simulink library "vmc"  (R2021b)
settings: Solver=VariableStepAuto  StartTime=0.0  StopTime=10.0  RelTol=1e-3
undefined symbols (not defined in the file): AVMC_ACCDeltaTqGradeGn_X_deg, AVMC_ACCDeltaTqIGain4OVRD_X_kph, AVMC_ACCDeltaTqIGain4OVRD_Y_mps2, AVMC_ACCDeltaTqIGain_X_kph, AVMC_ACCDeltaTqIGain_Y_mps2, AVMC_ACCDeltaTqPGain_X_kph, AVMC_ACCDeltaTqPGain_Y_kph, AVMC_ACCGradeofst_X_G, AVMC_ACCGradeofst_Y_pct, AVMC_ACCLoSpdTqLoLim4JP_X_kph, AVMC_ACCLoSpdTqLoLim4JP_Y_deg, AVMC_ACCLoSpdTqLowerLim_X_kph, AVMC_ACCLoSpdTqLowerLim_Y_deg, AVMC_ACCReqAccelGain_X_mps2, AVMC_ACCReqAccelGain_Y_enum, AVMC_ADSPosGFBDeltaTq_X_kph, AVMC_ADSPosGFBDeltaTq_Y_mps2, AVMC_AggressJerkPCT4AT_X_kph, AVMC_AggressJerkPCT_X_kph, AVMC_AggressLimitPCT4AT_X_kph, AVMC_AggressLimitPCT_X_kph, AVMC_DECGradeofst_X_G, AVMC_DECGradeofst_Y_pct, AVMC_DISCDeltaTqIGain_X_kph, AVMC_DISCDeltaTqIGain_Y_mps2, AVMC_DISCDeltaTqPGain_X_kph, AVMC_DISCDeltaTqPGain_Y_kph, AVMC_EPSForceSelect_X_enum, AVMC_EPSForceSelect_Y_enum, AVMC_EPSForceSelectD21_X_enum, AVMC_EPSForceSelectD21_Y_enum, AVMC_ESCRegenOut_X_kph, AVMC_ESCRegenOut_Y_Deg, AVMC_ESCRegenOutEnSpd_X_Deg, AVMC_EstPitchSlopeTs_X_kph, AVMC_GradeCompFlt_X_kph, AVMC_GyroYBandLo_X_Gps, AVMC_HoldResTq_X_kph, AVMC_ISOAccLimit_X_mps, AVMC_ISODecLimit_X_mps, AVMC_ISOJerk_X_mps, AVMC_LatESCRegenOut_X_kph, AVMC_LatESCRegenOut_Y_Deg, AVMC_LongAccDeadZone_X_kph, AVMC_LongAccFiltTsforP2_X_Gps, AVMC_MCPresBaseTq_X_bar, AVMC_MSAPedalOvrd_X_kph, AVMC_MSASpdBand_X_kph, AVMC_MSATqDownEndTq_X_kph, AVMC_MSATqDownTime_X_kph, AVMC_NegZCHoldTq_X_kph, AVMC_OPDDisSlideRate_X_Deg, AVMC_OVRD2ActSR2FCMCMD_X_mps2, AVMC_PedalTqRWhlRatio_X_Nm, AVMC_PedalTqRWhlRatio_Y_gps, AVMC_PedalTqRWhlSlipGain_X_rat, AVMC_PedalTqRWhlSlipGain_Y_kph, AVMC_PedalTqRWhSTRGGain_X_deg, AVMC_PedalTqRWhSTRGGain_Y_kph, AVMC_PosZCHoldTq_X_kph ... (+593)
libraries: hcu_lib x143, simulink x96, tqr x4, $bdroot x1, simulink_extras x1
(part 5 of 17)

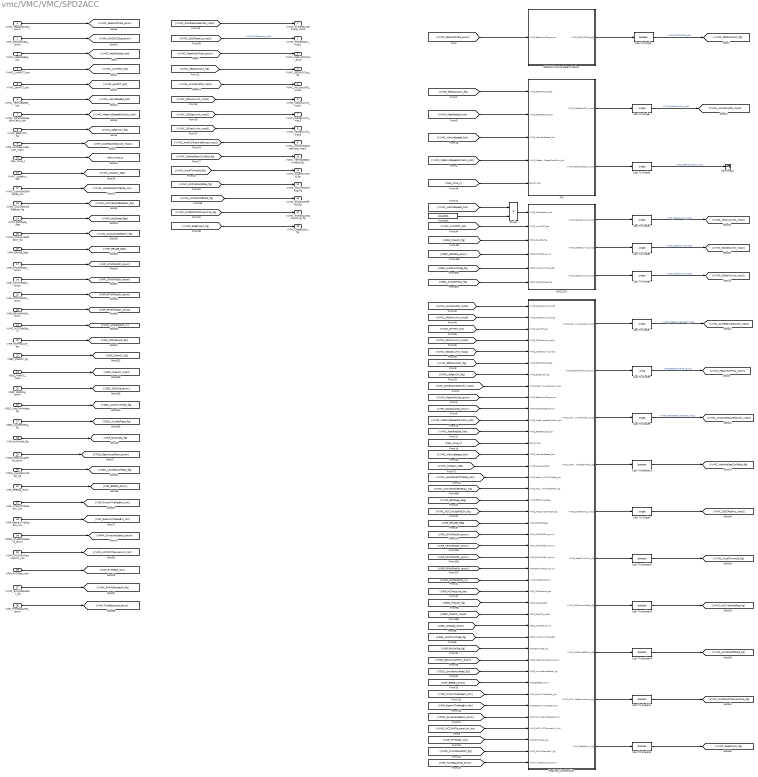
== system vmc/VMC/VMC/SPD2ACC ==
  VVMC_FeatArbitrSta_enum : Inport
  VINP_ADASACCSta_enum : Inport  Port=2
  VVMC_FeatReqSpd_kph : Inport  Port=3
  VVMC_LimitPCT_pct : Inport  Port=4
  VVMC_JerkPCT_pct : Inport  Port=5
  VVMC_VehicleSpeed_kph : Inport  Port=6
  VVMC_MeterIndSpeedForCalcu_kph : Inport  Port=7
  VVMC_SafetyCtrl_flg : Inport  Port=8
  VINP_ACCRequiredAccel_mps2 : Inport  Port=9
  task_time_s : Inport  Port=10
  VVMC_LongAcc_Gps : Inport  Port=11
  VVMC_LastADASWhlTqReq_Nm : Inport  Port=12
  VVMC_ACCVehHoldReqRaw_flg : Inport  Port=13
  VVMC_EstSlope_Deg : Inport  Port=14
  VVMC_ACCLowSpdTqCtrl_flg : Inport  Port=15
  VINP_GRADE_Deg : Inport  Port=16
  VINP_LFWhlRotDir_enum : Inport  Port=17
  VINP_LRWhlRotDir_enum : Inport  Port=18
  VINP_RFWhlRotDir_enum : Inport  Port=19
  VINP_RRWhlRotDir_enum : Inport  Port=20
  VVMC_ACCObjDist_m : Inport  Port=21
  VINP_MCPressure_bar : Inport  Port=22
  VDSC_PreACC_flg : Inport  Port=23
  VDSC_PreACC_mps2 : Inport  Port=24
  VDSC_DISCSta_enum : Inport  Port=25
  VDSC_AutoTurnMode_flg : Inport  Port=26
  VDSC_AccDecResp_flg : Inport  Port=27
  VINP_BrkSwSta_flg : Inport  Port=28
  VTQD_GearActualPosn_enum : Inport  Port=29
  VTQD_LowIdleAccPedal_flg : Inport  Port=30
  VINP_EPBSta_enum : Inport  Port=31
  VINP_FrntAxlTrqReqBrk_Nm : Inport  Port=32
  VINP_RearAxlTrqReqBrk_Nm : Inport  Port=33
  VPMM_DrivetrainSelect_enum : Inport  Port=34
  VVMC_ACCWhlTqLowerLim_Nm : Inport  Port=35
  VINP_RrTMSpd_rpm : Inport  Port=36
  VVMC_RrWhlStandstill_flg : Inport  Port=37
  VINP_TimeGapLevel_enum : Inport  Port=38
  Cast To Boolean{1..4} (4 alike) : DataTypeConversion  OutDataTypeStr=boolean
  Cast To Single : DataTypeConversion  OutDataTypeStr=boolean
  Cast To Single{1..7,9} (8 alike) : DataTypeConversion  OutDataTypeStr=single
  Cast To Single10 : DataTypeConversion  OutDataTypeStr=boolean
  Cast To Single11 : DataTypeConversion  OutDataTypeStr=boolean
  Cast To Single8 : DataTypeConversion  OutDataTypeStr=uint8
  Constant : Constant  Value=KPH2MPS
  Divide : Product  Inputs=**
  ISO22179 : Subsystem
  PID : Subsystem
  Required_Acceleration : Subsystem
  SPD2ACC Active Determination : Subsystem
  Terminator : Terminator
  VVMC_ACCRequiredAccel_mps2 : Outport
  VVMC_DISCReqAcc_mps2 : Outport  Port=2
  VVMC_FeatArbitrFinal_enum : Outport  Port=3
  VVMC_SPD2ACCAct_flg : Outport  Port=4
  VVMC_AccCalcuPID_mps2 : Outport  Port=5
  VVMC_ISOAccLimit_mps2 : Outport  Port=6
  VVMC_ISODecLimit_mps2 : Outport  Port=7
  VVMC_ISOJerkLimit_mps3 : Outport  Port=8
  VVMC_ActACCRequiredAccel_mps2 : Outport  Port=9
  VVMC_VehHoldDecCtrlHEnd_flg : Outport  Port=10
  VVMC_AccelTurnHold_flg : Outport  Port=11
  VVMC_ACCVehHoldReq_flg : Outport  Port=12
  VVMC_ACCShutOffHold_flg : Outport  Port=13
  VVMC_OVRD2ActRampActive_flg : Outport  Port=14
  VVMC_ReqBrkJoin_flg : Outport  Port=15
  wires:
  [VPMM_DrivetrainSelect_enum] -> Required_Acceleration/37(VPMM_DrivetrainSelect_enum)
  VPMM_DrivetrainSelect_enum/1 -> [VPMM_DrivetrainSelect_enum]
  [VINP_FrntAxlTrqReqBrk_Nm] -> Required_Acceleration/35(VINP_FrntAxlTrqReqBrk_Nm)
  [VINP_RearAxlTrqReqBrk_Nm] -> Required_Acceleration/36(VINP_RearAxlTrqReqBrk_Nm)
  VINP_RearAxlTrqReqBrk_Nm/1 -> [VINP_RearAxlTrqReqBrk_Nm]
  VINP_FrntAxlTrqReqBrk_Nm/1 -> [VINP_FrntAxlTrqReqBrk_Nm]
  [task_time_s] -> PID/5(task_time_s)
  [VVMC_OVRD2ActRampActive_flg] -> VVMC_OVRD2ActRampActive_flg/1
  Required_Acceleration/9(VVMC_OVRD2ActRampActive_flg) -> Cast To Single11/1
  Cast To Single11/1 -> [VVMC_OVRD2ActRampActive_flg]
  [VVMC_ACCShutOffHold_flg] -> VVMC_ACCShutOffHold_flg/1
  [VVMC_ACCVehHoldReq_flg] -> VVMC_ACCVehHoldReq_flg/1
  [VVMC_AccelTurnHold_flg] -> VVMC_AccelTurnHold_flg/1
  Cast To Boolean4/1 -> [VVMC_ACCShutOffHold_flg]
  Cast To Boolean3/1 -> [VVMC_ACCVehHoldReq_flg]
  Cast To Boolean2/1 -> [VVMC_AccelTurnHold_flg]
  Required_Acceleration/6(VVMC_AccelTurnHold_flg) -> Cast To Boolean2/1
  Required_Acceleration/7(VVMC_ACCVehHoldReq_flg) -> Cast To Boolean3/1
  Required_Acceleration/8(VVMC_ACCShutOffHold_flg) -> Cast To Boolean4/1
  VTQD_GearActualPosn_enum/1 -> [VTQD_GearActualPosn_enum]
  VINP_EPBSta_enum/1 -> [VINP_EPBSta_enum]
  VINP_BrkSwSta_flg/1 -> [VINP_BrkSwSta_flg]
  VTQD_LowIdleAccPedal_flg/1 -> [VTQD_LowIdleAccPedal_flg]
  [VINP_EPBSta_enum] -> Required_Acceleration/34(VINP_EPBSta_enum)
  [VTQD_LowIdleAccPedal_flg] -> Required_Acceleration/33(VTQD_LowIdleAccPedal_flg)
  [VTQD_GearActualPosn_enum] -> Required_Acceleration/32(VTQD_GearActualPosn_enum)
  [VINP_BrkSwSta_flg] -> Required_Acceleration/31(VINP_BrkSwSta_flg)
  VDSC_PreACC_mps2/1 -> [VDSC_PreACC_mps2]
  VDSC_PreACC_flg/1 -> [VDSC_PreACC_flg]
  VDSC_DISCSta_enum/1 -> [VDSC_DISCSta_enum]
  VDSC_AutoTurnMode_flg/1 -> [VDSC_AutoTurnMode_flg]
  VDSC_AccDecResp_flg/1 -> [VDSC_AccDecResp_flg]
  [VDSC_AutoTurnMode_flg] -> Required_Acceleration/30(VDSC_AutoTurnMode_flg)
  [VDSC_DISCSta_enum] -> Required_Acceleration/29(VDSC_DISCSta_enum)
  [VDSC_PreACC_mps2] -> Required_Acceleration/28(VDSC_PreACC_mps2)
  [VDSC_PreACC_flg] -> Required_Acceleration/27(VDSC_PreACC_flg)
  [VDSC_AccDecResp_flg] -> ISO22179/6(VDSC_AccDecResp_flg)
  [VDSC_AutoTurnMode_flg] -> ISO22179/5(VDSC_AutoTurnMode_flg)
  [VDSC_DISCSta_enum] -> ISO22179/4(VDSC_DISCSta_enum)
  [VDSC_PreACC_flg] -> ISO22179/3(VDSC_PreACC_flg)
  Constant/1 -> Divide/2
  [VVMC_VehicleSpeed_kph] -> Divide/1
  Divide/1 -> ISO22179/1(VVMC_VehSpeed_mps)
  [VVMC_FeatReqSpd_kph] -> PID/2(VVMC_FeatReqSpd_kph)
  Cast To Single3/1 -> [VVMC_DISCReqAcc_mps2]
  Required_Acceleration/5(VVMC_DISCReqAcc_mps2) -> Cast To Single3/1
  [VINP_MCPressure_bar] -> Required_Acceleration/26(VINP_MCPressure_bar)
  VINP_MCPressure_bar/1 -> [VINP_MCPressure_bar]
  [VVMC_ACCObjDist_m] -> Required_Acceleration/25(VVMC_ACCObjDist_m)
  VVMC_ACCObjDist_m/1 -> [VVMC_ACCObjDist_m]
  [VINP_LFWhlRotDir_enum] -> Required_Acceleration/21(VINP_LFWhlRotDir_enum)
  [VINP_LRWhlRotDir_enum] -> Required_Acceleration/22(VINP_LRWhlRotDir_enum)
  [VINP_RFWhlRotDir_enum] -> Required_Acceleration/23(VINP_RFWhlRotDir_enum)
  [VINP_RRWhlRotDir_enum] -> Required_Acceleration/24(VINP_RRWhlRotDir_enum)
  VINP_RRWhlRotDir_enum/1 -> [VINP_RRWhlRotDir_enum]
  VINP_LFWhlRotDir_enum/1 -> [VINP_LFWhlRotDir_enum]
  VINP_RFWhlRotDir_enum/1 -> [VINP_RFWhlRotDir_enum]
  VINP_LRWhlRotDir_enum/1 -> [VINP_LRWhlRotDir_enum]
  [VINP_GRADE_Deg] -> Required_Acceleration/20(VINP_GRADE_Deg)
  VINP_GRADE_Deg/1 -> [VINP_GRADE_Deg]
  [VVMC_ACCLowSpdTqCtrl_flg] -> Required_Acceleration/19(VVMC_ACCLowSpdTqCtrl_flg)
  VVMC_ACCLowSpdTqCtrl_flg/1 -> [VVMC_ACCLowSpdTqCtrl_flg]
  [VVMC_VehHoldDecCtrlHEnd_flg] -> VVMC_VehHoldDecCtrlHEnd_flg/1
  Cast To Boolean1/1 -> [VVMC_VehHoldDecCtrlHEnd_flg]
  Required_Acceleration/4(VVMC_VehHoldDecCtrlHEnd_flg) -> Cast To Boolean1/1
  [VVMC_EstSlope_Deg] -> Required_Acceleration/18(VVMC_EstSlope_Deg)
  VVMC_EstSlope_Deg/1 -> [VVMC_EstSlope_Deg]
  [VVMC_ACCVehHoldReqRaw_flg] -> Required_Acceleration/17(VVMC_ACCVehHoldReqRaw_flg)
  VVMC_ACCVehHoldReqRaw_flg/1 -> [VVMC_ACCVehHoldReqRaw_flg]
  [VVMC_ActACCRequiredAccel_mps2] -> VVMC_ActACCRequiredAccel_mps2/1
  VVMC_LastADASWhlTqReq_Nm/1 -> [VVMC_LastADASWhlTqReq_Nm]
  Required_Acceleration/3(VVMC_ActACCRequiredAccel_mps2) -> Cast To Single9/1
  Cast To Single9/1 -> [VVMC_ActACCRequiredAccel_mps2]  "VVMC_ActACCRequiredAccel_mps2"
  [VVMC_LastADASWhlTqReq_Nm] -> Required_Acceleration/16(VVMC_LastADASWhlTqReq_Nm)
  VVMC_LongAcc_Gps/1 -> [VVMC_LongAcc_Gps]
  [VVMC_LongAcc_Gps] -> Required_Acceleration/15(VVMC_LongAcc_Gps)
  [VVMC_VehicleSpeed_kph] -> Required_Acceleration/14(VVMC_VehicleSpeed_kph)
  [VVMC_ISODecLimit_mps2] -> Required_Acceleration/5(VVMC_ISODecLimit_mps2)
  [VVMC_ISOAccLimit_mps2] -> Required_Acceleration/4(VVMC_ISOAccLimit_mps2)
  [VVMC_AccCalcuPID_mps2] -> Required_Acceleration/1(VVMC_AccCalcuPID_mps2)
  [VVMC_ISOJerkLimit_mps3] -> Required_Acceleration/2(VVMC_ISOJerkLimit_mps3)
  [VVMC_JerkPCT_pct] -> Required_Acceleration/3(VVMC_JerkPCT_pct)
  VVMC_FeatReqSpd_kph/1 -> [VVMC_FeatReqSpd_kph]
  VVMC_JerkPCT_pct/1 -> [VVMC_JerkPCT_pct]
  VVMC_LimitPCT_pct/1 -> [VVMC_LimitPCT_pct]
  VVMC_MeterIndSpeedForCalcu_kph/1 -> [VVMC_MeterIndSpeedForCalcu_kph]
  VVMC_FeatArbitrSta_enum/1 -> [VVMC_FeatArbitrSta_enum]
  [VVMC_FeatArbitrSta_enum] -> SPD2ACC Active Determination/1(VVMC_FeatArbitrSta_enum)
  SPD2ACC Active Determination/1(VVMC_SPD2ACCAct_flg) -> Cast To Single/1
  [VVMC_LimitPCT_pct] -> ISO22179/2(VVMC_LimitPCT_pct)
  ISO22179/1(VVMC_ISOAccLimit_mps2) -> Cast To Single4/1
  ISO22179/2(VVMC_ISODecLimit_mps2) -> Cast To Single5/1
  ISO22179/3(VVMC_ISOJerkLimit_mps3) -> Cast To Single6/1
  [VVMC_SPD2ACCAct_flg] -> PID/1(VVMC_SPD2ACCAct_flg)
  [VVMC_MeterIndSpeedForCalcu_kph] -> PID/4(VVMC_MeterIndSpeedForCalcu_kph)
  PID/1(VVMC_AccCalcuPID_mps2) -> Cast To Single1/1
  PID/2(VVMC_MeterSpdCalcu_mps) -> Cast To Single2/1
  [VVMC_SPD2ACCAct_flg] -> Required_Acceleration/6(VVMC_SPD2ACCAct_flg)
  Required_Acceleration/1("VVMC_ACCRequiredAccel_mps2 ") -> Cast To Single7/1
  [VVMC_ACCRequiredAccel_mps2] -> VVMC_ACCRequiredAccel_mps2/1
  Cast To Single/1 -> [VVMC_SPD2ACCAct_flg]  "VVMC_SPD2ACCAct_flg"
  Cast To Single1/1 -> [VVMC_AccCalcuPID_mps2]  "VVMC_AccCalcuPID_mps2"
  Cast To Single2/1 -> Terminator/1  "VVMC_MeterSpdCalcu_mps"
  Cast To Single4/1 -> [VVMC_ISOAccLimit_mps2]  "VVMC_ISOAccLimit_mps2"
  Cast To Single5/1 -> [VVMC_ISODecLimit_mps2]  "VVMC_ISODecLimit_mps2"
  Cast To Single6/1 -> [VVMC_ISOJerkLimit_mps3]  "VVMC_ISOJerkLimit_mps3"
  Cast To Single7/1 -> [VVMC_ACCRequiredAccel_mps2]  "VVMC_ACCRequiredAccel_mps2"
  [VVMC_SafetyCtrl_flg] -> Required_Acceleration/7(VVMC_SafetyCtrl_flg)
  VVMC_SafetyCtrl_flg/1 -> [VVMC_SafetyCtrl_flg]
  VINP_ACCRequiredAccel_mps2/1 -> [VINP_ACCRequiredAccel_mps2]
  [VINP_ACCRequiredAccel_mps2] -> Required_Acceleration/8(VINP_ACCRequiredAccel_mps2)
  [VVMC_FeatArbitrSta_enum] -> Required_Acceleration/9(VVMC_FeatArbitrSta_enum)
  Required_Acceleration/2(VVMC_FeatArbitrFinal_enum) -> Cast To Single8/1
  Cast To Single8/1 -> [VVMC_FeatArbitrFinal_enum]  "VVMC_FeatArbitrFinal_enum"
  [VVMC_FeatArbitrFinal_enum] -> VVMC_FeatArbitrFinal_enum/1
  [VVMC_DISCReqAcc_mps2] -> VVMC_DISCReqAcc_mps2/1  "VVMC_DISCReqAcc_mps2"
  VINP_ADASACCSta_enum/1 -> [VINP_ADASACCSta_enum]
  [VINP_ADASACCSta_enum] -> Required_Acceleration/10(VINP_ADASACCSta_enum)
  [VVMC_MeterIndSpeedForCalcu_kph] -> Required_Acceleration/11(VVMC_MeterIndSpeedForCalcu_kph)
  [VVMC_FeatReqSpd_kph] -> Required_Acceleration/12(VVMC_FeatReqSpd_kph)
  [VVMC_SPD2ACCAct_flg] -> VVMC_SPD2ACCAct_flg/1
  [VVMC_AccCalcuPID_mps2] -> VVMC_AccCalcuPID_mps2/1
  [VVMC_ISOAccLimit_mps2] -> VVMC_ISOAccLimit_mps2/1
  [VVMC_ISODecLimit_mps2] -> VVMC_ISODecLimit_mps2/1
  [VVMC_ISOJerkLimit_mps3] -> VVMC_ISOJerkLimit_mps3/1
  VVMC_VehicleSpeed_kph/1 -> [VVMC_VehicleSpeed_kph]
  [VVMC_VehicleSpeed_kph] -> PID/3(VVMC_VehicleSpeed_kph)
  task_time_s/1 -> [task_time_s]
  [task_time_s] -> Required_Acceleration/13(task_time_s)
  Required_Acceleration/10(VVMC_ReqBrkJoin_flg) -> Cast To Single10/1
  Cast To Single10/1 -> [VVMC_ReqBrkJoin_flg]
  [VVMC_ReqBrkJoin_flg] -> VVMC_ReqBrkJoin_flg/1
  VVMC_ACCWhlTqLowerLim_Nm/1 -> [VVMC_ACCWhlTqLowerLim_Nm]
  [VVMC_ACCWhlTqLowerLim_Nm] -> Required_Acceleration/38(VVMC_ACCWhlTqLowerLim_Nm)
  [VINP_RrTMSpd_rpm] -> Required_Acceleration/39(VINP_RrTMSpd_rpm)
  VINP_RrTMSpd_rpm/1 -> [VINP_RrTMSpd_rpm]
  VVMC_RrWhlStandstill_flg/1 -> [VVMC_RrWhlStandstill_flg]
  [VVMC_RrWhlStandstill_flg] -> Required_Acceleration/40(VVMC_RrWhlStandstill_flg)
  VINP_TimeGapLevel_enum/1 -> [VINP_TimeGapLevel_enum]
  [VINP_TimeGapLevel_enum] -> Required_Acceleration/41(VINP_TimeGapLevel_enum)

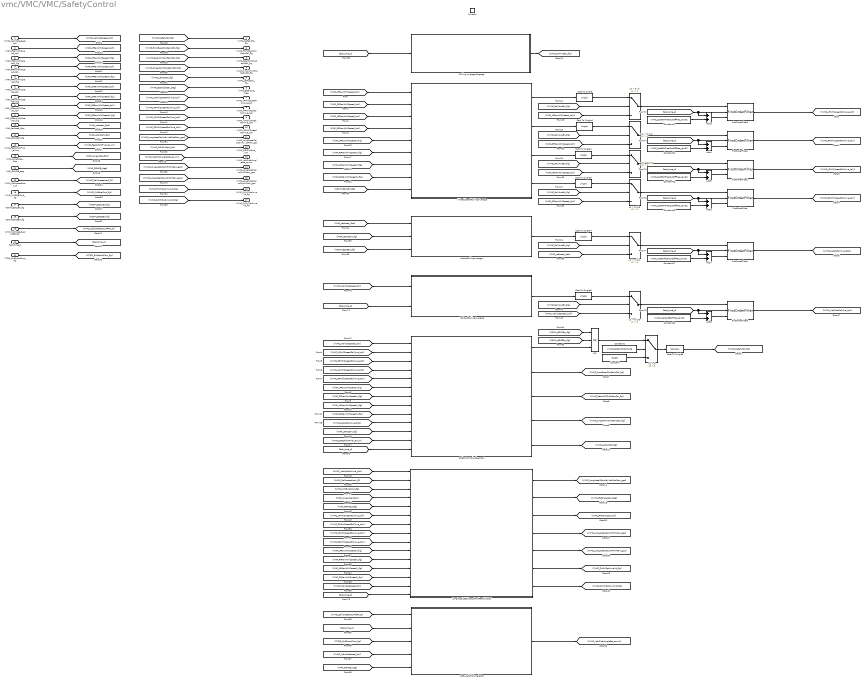
== system vmc/VMC/VMC/SafetyControl ==
  VVMC_VehicleSpeed_kph : Inport
  VINP_LFRawWhlSpeed_kph : Inport  Port=2
  VINP_LFRawWhlSpeedV_flg : Inport  Port=3
  VINP_RFRawWhlSpeed_kph : Inport  Port=4
  VINP_RFRawWhlSpeedV_flg : Inport  Port=5
  VINP_LRRawWhlSpeed_kph : Inport  Port=6
  VINP_LRRawWhlSpeedV_flg : Inport  Port=7
  VINP_RRRawWhlSpeed_kph : Inport  Port=8
  VINP_RRRawWhlSpeedV_flg : Inport  Port=9
  VINP_LatAccel_Gps : Inport  Port=10
  VINP_LatAccelV_flg : Inport  Port=11
  VVMC_FeatArbitrFinal_enum : Inport  Port=12
  VINP_LongAccel_Gps : Inport  Port=13
  VINP_GRADE_deg : Inport  Port=14
  VVMC_CalibratedAccX_G : Inport  Port=15
  VVMC_IMUEnaCmd_flg : Inport  Port=16
  VDDM_ESC1Err_flg : Inport  Port=17
  VDDM_ESC5Err_flg : Inport  Port=18
  VVMC_CalibratedAccXAftRA_G : Inport  Port=19
  task_time_s : Inport  Port=20
  VTQD_ExtDoorAllow_flg : Inport  Port=21
  function : TriggerPort  TriggerType=function-call  VariantControl=(inherit)
  ADB_VehPitchAngleSta : Subsystem
  Add{3..8} (6 alike) : Sum
  Cast To Single{,1..4,8} (6 alike) : DataTypeConversion  OutDataTypeStr=single
  Cast To Single5 : DataTypeConversion  OutDataTypeStr=boolean
  Constant : Constant  Value=FALSE
  Constant1 : Constant  Value=KVMC_SafetyCtrlSWC_flg
  Constant{11..13,15} (4 alike) : Constant  Value=KVMC_SpdBWFilterCutOffFreq_raw32
  Constant17 : Constant  Value=KVMC_AccBWFilterCutOffFreq_raw32
  Constant23 : Constant  Value=KVMC_VehSpdBWFilter_raw32
  FirstOrderFilter{,1..4,6} (6 alike) : hcu_lib/Basic_Blocks/FirstOrderFilter
  LatAccRollingAverage : Subsystem
  LongAccel_EstSlope_FrontRearSlipSpd : Subsystem
  OR : Logic  Operator=OR  Inputs=3  AllPortsSameDT=off  OutDataTypeStr=boolean
  Rolling Average Engage : Subsystem
  SafetyControlJudgement : Subsystem
  VehSpdRollingAverage : Subsystem
  WheelSpeedRollingAverage : Subsystem
  u2 > 0 : Switch  Criteria=u2 > Threshold
  u2 > 0 (1){,1..4,6} (6 alike) : Switch  Criteria=u2 > Threshold
  VVMC_SafetyCtrl_flg : Outport
  VVMC_FrontRearSlipRatioCtrl_flg : Outport  Port=2
  VVMC_RearWhlSlipRatioCtrl_flg : Outport  Port=3
  VVMC_SingleWhlSlipRatioCtrl_flg : Outport  Port=4
  VVMC_LatAccCtrl_flg : Outport  Port=5
  VVMC_EstSlope_Deg : Outport  Port=6
  VVMC_LFWhlSpeedRollAve_kph : Outport  Port=7
  VVMC_RFWhlSpeedRollAve_kph : Outport  Port=8
  VVMC_LRWhlSpeedRollAve_kph : Outport  Port=9
  VVMC_RRWhlSpeedRollAve_kph : Outport  Port=10
  VVMC_LongAccelCalcuByVehSpdRaw_gps : Outport  Port=11
  VVMC_FrRrSlipSpd_kph : Outport  Port=12
  VVMC_VehPitchAngleSta_enum : Outport  Port=13
  VVMC_LongAccelCalcuFrWhlRaw_gps : Outport  Port=14
  VVMC_LongAccelCalcuRrWhlRaw_gps : Outport  Port=15
  VVMC_FrWhlSpdInvalid_flg : Outport  Port=16
  VVMC_RrWhlSpdInvalid_flg : Outport  Port=17
  wires:
  [VVMC_VehPitchAngleSta_enum] -> VVMC_VehPitchAngleSta_enum/1
  VTQD_ExtDoorAllow_flg/1 -> [VTQD_ExtDoorAllow_flg]
  task_time_s/1 -> [task_time_s]
  VVMC_CalibratedAccXAftRA_G/1 -> [VVMC_CalibratedAccXAftRA_G]
  OR/1 -> u2 > 0/1
  [VDDM_ESC1Err_flg] -> OR/1
  [VDDM_ESC5Err_flg] -> OR/2
  [VDDM_ESC5Err_flg] -> LatAccRollingAverage/3(VDDM_ESC5Err_flg)
  [VDDM_ESC1Err_flg] -> WheelSpeedRollingAverage/9(VDDM_ESC1Err_flg)
  VDDM_ESC5Err_flg/1 -> [VDDM_ESC5Err_flg]
  VDDM_ESC1Err_flg/1 -> [VDDM_ESC1Err_flg]
  [VINP_LatAccelV_flg] -> LatAccRollingAverage/2(VINP_LatAccelV_flg)
  [VINP_RRRawWhlSpeedV_flg] -> WheelSpeedRollingAverage/8(VINP_RRRawWhlSpeedV_flg)
  [VINP_LRRawWhlSpeedV_flg] -> WheelSpeedRollingAverage/7(VINP_LRRawWhlSpeedV_flg)
  [VINP_RFRawWhlSpeedV_flg] -> WheelSpeedRollingAverage/6(VINP_RFRawWhlSpeedV_flg)
  [VINP_LFRawWhlSpeedV_flg] -> WheelSpeedRollingAverage/5(VINP_LFRawWhlSpeedV_flg)
  VVMC_IMUEnaCmd_flg/1 -> [VVMC_IMUEnaCmd_flg]
  VVMC_CalibratedAccX_G/1 -> [VVMC_CalibratedAccX_G]
  [VVMC_FrRrSlipSpd_kph] -> VVMC_FrRrSlipSpd_kph/1
  [VVMC_LongAccelCalcuByVehSpdRaw_gps] -> VVMC_LongAccelCalcuByVehSpdRaw_gps/1  "VVMC_LongAccelCalcuByVehSpd_gps"
  VehSpdRollingAverage/1(VVMC_VehSpdRollAveRaw_kph) -> Cast To Single8/1
  FirstOrderFilter6/1 -> [VVMC_VehSpdRollAve_kph]  "VVMC_VehSpdRollAve_kph"
  [VVMC_RollAveEn_flg] -> u2 > 0 (1)6/2
  [VVMC_VehicleSpeed_kph] -> u2 > 0 (1)6/3
  u2 > 0 (1)6/1 -> FirstOrderFilter6/1
  Cast To Single8/1 -> u2 > 0 (1)6/1
  [task_time_s] -> FirstOrderFilter6/2, Add8/1
  Constant23/1 -> Add8/2
  Add8/1 -> FirstOrderFilter6/3
  [VVMC_VehicleSpeed_kph] -> VehSpdRollingAverage/1(VVMC_VehicleSpeed_kph)
  [VVMC_LFWhlSpeedRollAve_kph] -> VVMC_LFWhlSpeedRollAve_kph/1  "VVMC_LFWhlSpeedRollAve_kph"
  [VVMC_RFWhlSpeedRollAve_kph] -> VVMC_RFWhlSpeedRollAve_kph/1  "VVMC_RFWhlSpeedRollAve_kph"
  [VVMC_LRWhlSpeedRollAve_kph] -> VVMC_LRWhlSpeedRollAve_kph/1  "VVMC_LRWhlSpeedRollAve_kph"
  [VVMC_RRWhlSpeedRollAve_kph] -> VVMC_RRWhlSpeedRollAve_kph/1  "VVMC_RRWhlSpeedRollAve_kph"
  [VVMC_EstSlopeCal_Deg] -> VVMC_EstSlope_Deg/1
  VINP_GRADE_deg/1 -> [VINP_GRADE_deg]
  VINP_LongAccel_Gps/1 -> [VINP_LongAccel_Gps]
  u2 > 0 (1)4/1 -> FirstOrderFilter4/1
  [task_time_s] -> Add7/1, FirstOrderFilter4/2
  Constant17/1 -> Add7/2
  Add7/1 -> FirstOrderFilter4/3
  [VINP_LatAccel_Gps] -> u2 > 0 (1)4/3
  Cast To Single4/1 -> u2 > 0 (1)4/1
  [VVMC_RollAveEn_flg] -> u2 > 0 (1)4/2
  Add6/1 -> FirstOrderFilter/3
  Constant15/1 -> Add6/2
  Add5/1 -> FirstOrderFilter1/3
  Constant13/1 -> Add5/2
  Add4/1 -> FirstOrderFilter2/3
  Constant12/1 -> Add4/2
  Constant11/1 -> Add3/2
  Add3/1 -> FirstOrderFilter3/3
  [task_time_s] -> Add6/1, FirstOrderFilter/2
  [task_time_s] -> FirstOrderFilter1/2, Add5/1
  [task_time_s] -> Add4/1, FirstOrderFilter2/2
  [task_time_s] -> FirstOrderFilter3/2, Add3/1
  [VVMC_RollAveEn_flg] -> u2 > 0 (1)2/2
  Cast To Single3/1 -> u2 > 0 (1)3/1
  u2 > 0 (1)3/1 -> FirstOrderFilter/1
  Cast To Single1/1 -> u2 > 0 (1)1/1
  Cast To Single2/1 -> u2 > 0 (1)2/1
  [VVMC_RollAveEn_flg] -> u2 > 0 (1)1/2
  u2 > 0 (1)1/1 -> FirstOrderFilter2/1
  [VINP_RRRawWhlSpeed_kph] -> u2 > 0 (1)3/3
  Cast To Single/1 -> u2 > 0 (1)/1
  [VINP_LFRawWhlSpeed_kph] -> u2 > 0 (1)/3
  [VVMC_RollAveEn_flg] -> u2 > 0 (1)/2
  [VVMC_RollAveEn_flg] -> u2 > 0 (1)3/2
  [VINP_LRRawWhlSpeed_kph] -> u2 > 0 (1)2/3
  [VINP_RFRawWhlSpeed_kph] -> u2 > 0 (1)1/3
  u2 > 0 (1)/1 -> FirstOrderFilter3/1
  u2 > 0 (1)2/1 -> FirstOrderFilter1/1
  VINP_RFRawWhlSpeedV_flg/1 -> [VINP_RFRawWhlSpeedV_flg]
  Constant/1 -> u2 > 0/3
  FirstOrderFilter1/1 -> [VVMC_LRWhlSpeedRollAve_kph]  "VVMC_LRWhlSpeedRollAve_kph"
  [VVMC_RFWhlSpeedRollAve_kph] -> SafetyControlJudgement/3(VVMC_RFWhlSpeedRollAve_kph)
  VINP_RFRawWhlSpeed_kph/1 -> [VINP_RFRawWhlSpeed_kph]
  Cast To Single5/1 -> [VVMC_SafetyCtrl_flg]  "VVMC_SafetyCtrl_flg"
  [VVMC_FrontRearSlipRatioCtrl_flg] -> VVMC_FrontRearSlipRatioCtrl_flg/1
  [VVMC_LFWhlSpeedRollAve_kph] -> SafetyControlJudgement/2(VVMC_LFWhlSpeedRollAve_kph)
  FirstOrderFilter2/1 -> [VVMC_RFWhlSpeedRollAve_kph]  "VVMC_RFWhlSpeedRollAve_kph"
  [VVMC_SafetyCtrl_flg] -> VVMC_SafetyCtrl_flg/1
  VVMC_VehicleSpeed_kph/1 -> [VVMC_VehicleSpeed_kph]
  VINP_LRRawWhlSpeedV_flg/1 -> [VINP_LRRawWhlSpeedV_flg]
  [VVMC_VehicleSpeed_kph] -> SafetyControlJudgement/1(VVMC_VehicleSpeed_kph)
  VVMC_FeatArbitrFinal_enum/1 -> [VVMC_FeatArbitrFinal_enum]
  [VINP_LRRawWhlSpeedV_flg] -> SafetyControlJudgement/8(VINP_LRRawWhlSpeedV_flg)
  [VINP_RRRawWhlSpeedV_flg] -> SafetyControlJudgement/9(VINP_RRRawWhlSpeedV_flg)
  SafetyControlJudgement/1(VVMC_SafetyCtrl_flg) -> OR/3
  [VVMC_FeatArbitrFinal_enum] -> SafetyControlJudgement/12(VVMC_FeatArbitrFinal_enum)
  VINP_LFRawWhlSpeedV_flg/1 -> [VINP_LFRawWhlSpeedV_flg]
  [VINP_LFRawWhlSpeed_kph] -> WheelSpeedRollingAverage/1(VINP_LFRawWhlSpeed_kph)
  VINP_LatAccelV_flg/1 -> [VINP_LatAccelV_flg]
  SafetyControlJudgement/3(VVMC_RearWhlSlipRatioCtrl_flg) -> [VVMC_RearWhlSlipRatioCtrl_flg]
  WheelSpeedRollingAverage/3(VVMC_LRWhlSpeedRollAveRaw_kph) -> Cast To Single2/1
  [VVMC_RRWhlSpeedRollAve_kph] -> SafetyControlJudgement/5(VVMC_RRWhlSpeedRollAve_kph)
  [VINP_RRRawWhlSpeed_kph] -> WheelSpeedRollingAverage/4(VINP_RRRawWhlSpeed_kph)
  [VVMC_LRWhlSpeedRollAve_kph] -> SafetyControlJudgement/4(VVMC_LRWhlSpeedRollAve_kph)
  VINP_RRRawWhlSpeedV_flg/1 -> [VINP_RRRawWhlSpeedV_flg]
  [VVMC_RearWhlSlipRatioCtrl_flg] -> VVMC_RearWhlSlipRatioCtrl_flg/1
  u2 > 0/1 -> Cast To Single5/1
  FirstOrderFilter4/1 -> [VVMC_LatAccRollAve_Gps]  "VVMC_LatAccRollAve_Gps"
  VINP_LRRawWhlSpeed_kph/1 -> [VINP_LRRawWhlSpeed_kph]
  Constant1/1 -> u2 > 0/2
  [VINP_RFRawWhlSpeedV_flg] -> SafetyControlJudgement/7(VINP_RFRawWhlSpeedV_flg)
  [VVMC_LatAccCtrl_flg] -> VVMC_LatAccCtrl_flg/1
  SafetyControlJudgement/4(VVMC_SingleWhlSlipRatioCtrl_flg) -> [VVMC_SingleWhlSlipRatioCtrl_flg]
  WheelSpeedRollingAverage/1(VVMC_LFWhlSpeedRollAveRaw_kph) -> Cast To Single/1
  VINP_LatAccel_Gps/1 -> [VINP_LatAccel_Gps]
  LatAccRollingAverage/1(VVMC_LatAccRollAveRaw_Gps) -> Cast To Single4/1
  [VINP_LatAccel_Gps] -> LatAccRollingAverage/1(VINP_LatAccel_Gps)
  VINP_RRRawWhlSpeed_kph/1 -> [VINP_RRRawWhlSpeed_kph]
  [VINP_LFRawWhlSpeedV_flg] -> SafetyControlJudgement/6(VINP_LFRawWhlSpeedV_flg)
  [VINP_LatAccelV_flg] -> SafetyControlJudgement/11(VINP_LatAccelV_flg)
  FirstOrderFilter3/1 -> [VVMC_LFWhlSpeedRollAve_kph]  "VVMC_LFWhlSpeedRollAve_kph"
  WheelSpeedRollingAverage/2(VVMC_RFWhlSpeedRollAveRaw_kph) -> Cast To Single1/1
  [VINP_RFRawWhlSpeed_kph] -> WheelSpeedRollingAverage/2(VINP_RFRawWhlSpeed_kph)
  SafetyControlJudgement/5(VVMC_LatAccCtrl_flg) -> [VVMC_LatAccCtrl_flg]
  SafetyControlJudgement/2(VVMC_FrontRearSlipRatioCtrl_flg) -> [VVMC_FrontRearSlipRatioCtrl_flg]
  VINP_LFRawWhlSpeed_kph/1 -> [VINP_LFRawWhlSpeed_kph]
  [VVMC_SingleWhlSlipRatioCtrl_flg] -> VVMC_SingleWhlSlipRatioCtrl_flg/1
  [VVMC_LatAccRollAve_Gps] -> SafetyControlJudgement/10(VVMC_LatAccRollAve_Gps)
  FirstOrderFilter/1 -> [VVMC_RRWhlSpeedRollAve_kph]  "VVMC_RRWhlSpeedRollAve_kph"
  [VINP_LRRawWhlSpeed_kph] -> WheelSpeedRollingAverage/3(VINP_LRRawWhlSpeed_kph)
  WheelSpeedRollingAverage/4(VVMC_RRWhlSpeedRollAveRaw_kph) -> Cast To Single3/1
  Rolling Average Engage/1(VVMC_RollAveEn_flg) -> [VVMC_RollAveEn_flg]
  [VVMC_VehSpdRollAve_kph] -> LongAccel_EstSlope_FrontRearSlipSpd/1(VVMC_VehSpdRollAve_kph)
  [VVMC_CalibratedAccX_G] -> LongAccel_EstSlope_FrontRearSlipSpd/2(VVMC_CalibratedAccX_G)
  [VVMC_IMUEnaCmd_flg] -> LongAccel_EstSlope_FrontRearSlipSpd/3(VVMC_IMUEnaCmd_flg)
  [VINP_LongAccel_Gps] -> LongAccel_EstSlope_FrontRearSlipSpd/4(VINP_LongAccel_Gps)
  [VINP_GRADE_deg] -> LongAccel_EstSlope_FrontRearSlipSpd/5(VINP_GRADE_deg)
  [VVMC_LFWhlSpeedRollAve_kph] -> LongAccel_EstSlope_FrontRearSlipSpd/6(VVMC_LFWhlSpeedRollAve_kph)
  [VVMC_RFWhlSpeedRollAve_kph] -> LongAccel_EstSlope_FrontRearSlipSpd/7(VVMC_RFWhlSpeedRollAve_kph)
  [VVMC_LRWhlSpeedRollAve_kph] -> LongAccel_EstSlope_FrontRearSlipSpd/8(VVMC_LRWhlSpeedRollAve_kph)
  [VVMC_RRWhlSpeedRollAve_kph] -> LongAccel_EstSlope_FrontRearSlipSpd/9(VVMC_RRWhlSpeedRollAve_kph)
  [VINP_LFRawWhlSpeedV_flg] -> LongAccel_EstSlope_FrontRearSlipSpd/10(VINP_LFRawWhlSpeedV_flg)
  [VINP_RFRawWhlSpeedV_flg] -> LongAccel_EstSlope_FrontRearSlipSpd/11(VINP_RFRawWhlSpeedV_flg)
  [VINP_LRRawWhlSpeedV_flg] -> LongAccel_EstSlope_FrontRearSlipSpd/12(VINP_LRRawWhlSpeedV_flg)
  [VINP_RRRawWhlSpeedV_flg] -> LongAccel_EstSlope_FrontRearSlipSpd/13(VINP_RRRawWhlSpeedV_flg)
  LongAccel_EstSlope_FrontRearSlipSpd/1(VVMC_LongAccelCalcuByVehSpdRaw_gps) -> [VVMC_LongAccelCalcuByVehSpdRaw_gps]
  LongAccel_EstSlope_FrontRearSlipSpd/2(VVMC_EstSlopeCal_Deg) -> [VVMC_EstSlopeCal_Deg]
  LongAccel_EstSlope_FrontRearSlipSpd/3(VVMC_FrRrSlipSpd_kph) -> [VVMC_FrRrSlipSpd_kph]
  ADB_VehPitchAngleSta/1(VVMC_VehPitchAngleSta_enum) -> [VVMC_VehPitchAngleSta_enum]
  [VVMC_CalibratedAccXAftRA_G] -> ADB_VehPitchAngleSta/1(VVMC_CalibratedAccXAftRA_G)
  [task_time_s] -> ADB_VehPitchAngleSta/2(task_time_s)
  [VTQD_ExtDoorAllow_flg] -> ADB_VehPitchAngleSta/3(VTQD_ExtDoorAllow_flg)
  [VVMC_VehicleSpeed_kph] -> ADB_VehPitchAngleSta/4(VVMC_VehicleSpeed_kph)
  [VINP_GRADE_deg] -> ADB_VehPitchAngleSta/5(VINP_GRADE_deg)
  [VVMC_VehicleSpeed_kph] -> LongAccel_EstSlope_FrontRearSlipSpd/14(VVMC_VehicleSpeed_kph)
  [task_time_s] -> VehSpdRollingAverage/2(task_time_s)
  [task_time_s] -> LongAccel_EstSlope_FrontRearSlipSpd/15(task_time_s)
  [task_time_s] -> Rolling Average Engage/1(task_time_s)
  [task_time_s] -> SafetyControlJudgement/13(task_time_s)
  [VVMC_LongAccelCalcuRrWhlRaw_gps] -> VVMC_LongAccelCalcuRrWhlRaw_gps/1
  [VVMC_LongAccelCalcuFrWhlRaw_gps] -> VVMC_LongAccelCalcuFrWhlRaw_gps/1
  LongAccel_EstSlope_FrontRearSlipSpd/4(VVMC_LongAccelCalcuFrWhlRaw_gps) -> [VVMC_LongAccelCalcuFrWhlRaw_gps]
  LongAccel_EstSlope_FrontRearSlipSpd/5(VVMC_LongAccelCalcuRrWhlRaw_gps) -> [VVMC_LongAccelCalcuRrWhlRaw_gps]
  LongAccel_EstSlope_FrontRearSlipSpd/6(VVMC_FrWhlSpdInvalid_flg) -> [VVMC_FrWhlSpdInvalid_flg]
  LongAccel_EstSlope_FrontRearSlipSpd/7(VVMC_RrWhlSpdInvalid_flg) -> [VVMC_RrWhlSpdInvalid_flg]
  [VVMC_FrWhlSpdInvalid_flg] -> VVMC_FrWhlSpdInvalid_flg/1
  [VVMC_RrWhlSpdInvalid_flg] -> VVMC_RrWhlSpdInvalid_flg/1

== system vmc/VMC/VMC/Slide Rate  Calculation ==
  VINP_LFRawWhlSpeed_kph : Inport
  VINP_RFRawWhlSpeed_kph : Inport  Port=2
  VINP_LRRawWhlSpeed_kph : Inport  Port=3
  VINP_RRRawWhlSpeed_kph : Inport  Port=4
  VVMC_VehicleSpeed_kph : Inport  Port=5
  VINP_BrkPedalPos_pct : Inport  Port=6
  VINP_BrkSwSta_flg : Inport  Port=7
  VINP_LongAccel_Gps : Inport  Port=8
  VVMC_LongAcc_Gps : Inport  Port=9
  task_time_s : Inport  Port=10
  VTQD_AfterAvailableTqDemFr_Nm : Inport  Port=11
  VTQD_AfterAvailableTqDemRr_Nm : Inport  Port=12
  VTQD_EquivAccPedalSWSta_flg : Inport  Port=13
  VTQD_GearActualPosn_enum : Inport  Port=14
  VTQD_RegenMode_enum : Inport  Port=15
  VTQD_VehActSpd_kph : Inport  Port=16
  VVMC_EstSlope_Deg : Inport  Port=17
  4Wheel Calculation : Subsystem
  Alternative Wheel Slide Calculation : Subsystem
  Coordination : Subsystem
  Partial Wheel Calculation : Subsystem
  VVMC_RawWhlSpdSlideRate_pct : Outport
  VVMC_LFWhlSpdSlideRate_pct : Outport  Port=2
  VVMC_RFWhlSpdSlideRate_pct : Outport  Port=3
  VVMC_LRWhlSpdSlideRate_pct : Outport  Port=4
  VVMC_RRWhlSpdSlideRate_pct : Outport  Port=5
  VVMC_LF4WhlSpdSlideRate_pct : Outport  Port=6
  VVMC_RF4WhlSpdSlideRate_pct : Outport  Port=7
  VVMC_LR4WhlSpdSlideRate_pct : Outport  Port=8
  VVMC_RR4WhlSpdSlideRate_pct : Outport  Port=9
  VVMC_PredictVehSpd_kph : Outport  Port=10
  VVMC_4WhlSpdSlideRate_pct : Outport  Port=11
  VVMC_ActMaxSlideRate_pct : Outport  Port=12
  VVMC_ActLFSlideRate_pct : Outport  Port=13
  VVMC_ActRFSlideRate_pct : Outport  Port=14
  VVMC_ActLRSlideRate_pct : Outport  Port=15
  VVMC_ActRRSlideRate_pct : Outport  Port=16
  VVMC_AltLWhlSlideRate_pct : Outport  Port=17
  VVMC_AltRWhlSlideRate_pct : Outport  Port=18
  VVMC_AltWhlSlideRate_pct : Outport  Port=19
  wires:
  [VVMC_EstSlope_Deg] -> Coordination/23(VVMC_EstSlope_Deg)
  [VTQD_VehActSpd_kph] -> Coordination/21(VTQD_VehActSpd_kph)
  [VTQD_RegenMode_enum] -> Coordination/22(VTQD_RegenMode_enum)
  VTQD_VehActSpd_kph/1 -> [VTQD_VehActSpd_kph]
  VTQD_RegenMode_enum/1 -> [VTQD_RegenMode_enum]
  VVMC_EstSlope_Deg/1 -> [VVMC_EstSlope_Deg]
  [VINP_LongAccel_Gps] -> 4Wheel Calculation/11(VINP_LongAccel_Gps)
  VINP_LongAccel_Gps/1 -> [VINP_LongAccel_Gps]
  VTQD_GearActualPosn_enum/1 -> [VTQD_GearActualPosn_enum]
  [VTQD_GearActualPosn_enum] -> 4Wheel Calculation/10(VTQD_GearActualPosn_enum)
  [VVMC_RF4WhlSpdSlideRate_pct] -> Coordination/15(VVMC_RF4WhlSpdSlideRate_pct)
  Coordination/2(VVMC_ActLFSlideRate_pct) -> [VVMC_ActLFSlideRate_pct]
  Coordination/5(VVMC_ActRRSlideRate_pct) -> [VVMC_ActRRSlideRate_pct]
  Coordination/1(VVMC_ActMaxSlideRate_pct) -> [VVMC_ActMaxSlideRate_pct]
  [VINP_BrkPedalPos_pct] -> Coordination/3(VINP_BrkPedalPos_pct)
  [VVMC_RRWhlSpdSlideRate_pct] -> Coordination/12(VVMC_RRWhlSpdSlideRate_pct)
  [VVMC_LRWhlSpdSlideRate_pct] -> Coordination/11(VVMC_LRWhlSpdSlideRate_pct)
  [VINP_BrkSwSta_flg] -> Coordination/7(VINP_BrkSwSta_flg)
  [VVMC_PredictVehSpd_kph] -> Coordination/4(VVMC_PredictVehSpd_kph)
  Coordination/4(VVMC_ActLRSlideRate_pct) -> [VVMC_ActLRSlideRate_pct]
  [VTQD_AfterAvailableTqDemRr_Nm] -> Coordination/19(VTQD_AfterAvailableTqDemRr_Nm)
  [VVMC_RawWhlSpdSlideRate_pct] -> Coordination/8(VVMC_RawWhlSpdSlideRate_pct)
  Coordination/3(VVMC_ActRFSlideRate_pct) -> [VVMC_ActRFSlideRate_pct]
  [VVMC_VehicleSpeed_kph] -> Coordination/5(VVMC_VehicleSpeed_kph)
  [VVMC_4WhlSpdSlideRate_pct] -> Coordination/13(VVMC_4WhlSpdSlideRate_pct)
  [VVMC_AllWhlSkid_flg] -> Coordination/18(VVMC_AllWhlSkid_flg)
  [VTQD_EquivAccPedalSWSta_flg] -> Coordination/2(VTQD_EquivAccPedalSWSta_flg)
  [VVMC_RFWhlSpdSlideRate_pct] -> Coordination/10(VVMC_RFWhlSpdSlideRate_pct)
  [VVMC_AltWhlSlideRate_pct] -> Coordination/20(VVMC_AltWhlSlideRate_pct)
  [VTQD_AfterAvailableTqDemFr_Nm] -> Coordination/1(VTQD_AfterAvailableTqDemFr_Nm)
  [VVMC_LFWhlSpdSlideRate_pct] -> Coordination/9(VVMC_LFWhlSpdSlideRate_pct)
  [task_time_s] -> Coordination/6(task_time_s)
  [VVMC_LR4WhlSpdSlideRate_pct] -> Coordination/16(VVMC_LR4WhlSpdSlideRate_pct)
  [VVMC_RR4WhlSpdSlideRate_pct] -> Coordination/17(VVMC_RR4WhlSpdSlideRate_pct)
  [VVMC_LF4WhlSpdSlideRate_pct] -> Coordination/14(VVMC_LF4WhlSpdSlideRate_pct)
  4Wheel Calculation/6(VVMC_4WhlSpdSlideRate_pct) -> [VVMC_4WhlSpdSlideRate_pct]
  4Wheel Calculation/2(VVMC_RF4WhlSpdSlideRate_pct) -> [VVMC_RF4WhlSpdSlideRate_pct]
  [VINP_RFRawWhlSpeed_kph] -> 4Wheel Calculation/2(VINP_RFRawWhlSpeed_kph)
  [VINP_LFRawWhlSpeed_kph] -> 4Wheel Calculation/1(VINP_LFRawWhlSpeed_kph)
  [VINP_RRRawWhlSpeed_kph] -> 4Wheel Calculation/4(VINP_RRRawWhlSpeed_kph)
  [VINP_LRRawWhlSpeed_kph] -> 4Wheel Calculation/3(VINP_LRRawWhlSpeed_kph)
  4Wheel Calculation/5(VVMC_PredictVehSpd_kph) -> [VVMC_PredictVehSpd_kph]
  [VVMC_VehicleSpeed_kph] -> 4Wheel Calculation/7(VVMC_VehicleSpeed_kph)
  [VTQD_AfterAvailableTqDemFr_Nm] -> 4Wheel Calculation/8(VTQD_AfterAvailableTqDemFr_Nm)
  [VTQD_AfterAvailableTqDemRr_Nm] -> 4Wheel Calculation/9(VTQD_AfterAvailableTqDemRr_Nm)
  4Wheel Calculation/4(VVMC_RR4WhlSpdSlideRate_pct) -> [VVMC_RR4WhlSpdSlideRate_pct]
  [VVMC_LongAcc_Gps] -> 4Wheel Calculation/5(VVMC_LongAcc_Gps)
  4Wheel Calculation/7(VVMC_AllWhlSkid_flg) -> [VVMC_AllWhlSkid_flg]
  4Wheel Calculation/1(VVMC_LF4WhlSpdSlideRate_pct) -> [VVMC_LF4WhlSpdSlideRate_pct]
  [task_time_s] -> 4Wheel Calculation/6(task_time_s)
  4Wheel Calculation/3(VVMC_LR4WhlSpdSlideRate_pct) -> [VVMC_LR4WhlSpdSlideRate_pct]
  Partial Wheel Calculation/4(VVMC_LRWhlSpdSlideRate_pct) -> [VVMC_LRWhlSpdSlideRate_pct]
  [VTQD_AfterAvailableTqDemRr_Nm] -> Partial Wheel Calculation/6(VTQD_AfterAvailableTqDemRr_Nm)
  [VINP_RRRawWhlSpeed_kph] -> Partial Wheel Calculation/4(VINP_RRRawWhlSpeed_kph)
  [VINP_LFRawWhlSpeed_kph] -> Partial Wheel Calculation/1(VINP_LFRawWhlSpeed_kph)
  [VTQD_AfterAvailableTqDemFr_Nm] -> Partial Wheel Calculation/5(VTQD_AfterAvailableTqDemFr_Nm)
  [VINP_LRRawWhlSpeed_kph] -> Partial Wheel Calculation/3(VINP_LRRawWhlSpeed_kph)
  [VINP_RFRawWhlSpeed_kph] -> Partial Wheel Calculation/2(VINP_RFRawWhlSpeed_kph)
  Partial Wheel Calculation/1(VVMC_RawWhlSpdSlideRate_pct) -> [VVMC_RawWhlSpdSlideRate_pct]
  Partial Wheel Calculation/3(VVMC_RFWhlSpdSlideRate_pct) -> [VVMC_RFWhlSpdSlideRate_pct]
  Partial Wheel Calculation/5(VVMC_RRWhlSpdSlideRate_pct) -> [VVMC_RRWhlSpdSlideRate_pct]
  Partial Wheel Calculation/2(VVMC_LFWhlSpdSlideRate_pct) -> [VVMC_LFWhlSpdSlideRate_pct]
  [VVMC_AltWhlSlideRate_pct] -> VVMC_AltWhlSlideRate_pct/1
  [VVMC_AltRWhlSlideRate_pct] -> VVMC_AltRWhlSlideRate_pct/1
  [VVMC_AltLWhlSlideRate_pct] -> VVMC_AltLWhlSlideRate_pct/1
  Alternative Wheel Slide Calculation/3(VVMC_AltWhlSlideRate_pct) -> [VVMC_AltWhlSlideRate_pct]
  Alternative Wheel Slide Calculation/2(VVMC_AltRWhlSlideRate_pct) -> [VVMC_AltRWhlSlideRate_pct]
  Alternative Wheel Slide Calculation/1(VVMC_AltLWhlSlideRate_pct) -> [VVMC_AltLWhlSlideRate_pct]
  [VINP_RRRawWhlSpeed_kph] -> Alternative Wheel Slide Calculation/4(VINP_RRRawWhlSpeed_kph)
  [VINP_LRRawWhlSpeed_kph] -> Alternative Wheel Slide Calculation/3(VINP_LRRawWhlSpeed_kph)
  [VINP_RFRawWhlSpeed_kph] -> Alternative Wheel Slide Calculation/2(VINP_RFRawWhlSpeed_kph)
  [VINP_LFRawWhlSpeed_kph] -> Alternative Wheel Slide Calculation/1(VINP_LFRawWhlSpeed_kph)
  VTQD_AfterAvailableTqDemRr_Nm/1 -> [VTQD_AfterAvailableTqDemRr_Nm]
  VVMC_LongAcc_Gps/1 -> [VVMC_LongAcc_Gps]
  [VVMC_4WhlSpdSlideRate_pct] -> VVMC_4WhlSpdSlideRate_pct/1
  [VVMC_ActLFSlideRate_pct] -> VVMC_ActLFSlideRate_pct/1
  [VVMC_LRWhlSpdSlideRate_pct] -> VVMC_LRWhlSpdSlideRate_pct/1
  VINP_LFRawWhlSpeed_kph/1 -> [VINP_LFRawWhlSpeed_kph]
  [VVMC_RawWhlSpdSlideRate_pct] -> VVMC_RawWhlSpdSlideRate_pct/1
  [VVMC_LF4WhlSpdSlideRate_pct] -> VVMC_LF4WhlSpdSlideRate_pct/1
  VINP_LRRawWhlSpeed_kph/1 -> [VINP_LRRawWhlSpeed_kph]
  [VVMC_PredictVehSpd_kph] -> VVMC_PredictVehSpd_kph/1
  [VVMC_ActLRSlideRate_pct] -> VVMC_ActLRSlideRate_pct/1
  VVMC_VehicleSpeed_kph/1 -> [VVMC_VehicleSpeed_kph]
  VINP_RFRawWhlSpeed_kph/1 -> [VINP_RFRawWhlSpeed_kph]
  [VVMC_RR4WhlSpdSlideRate_pct] -> VVMC_RR4WhlSpdSlideRate_pct/1
  [VVMC_ActRFSlideRate_pct] -> VVMC_ActRFSlideRate_pct/1
  [VVMC_LR4WhlSpdSlideRate_pct] -> VVMC_LR4WhlSpdSlideRate_pct/1
  [VVMC_RFWhlSpdSlideRate_pct] -> VVMC_RFWhlSpdSlideRate_pct/1
  [VVMC_ActMaxSlideRate_pct] -> VVMC_ActMaxSlideRate_pct/1
  VINP_RRRawWhlSpeed_kph/1 -> [VINP_RRRawWhlSpeed_kph]
  task_time_s/1 -> [task_time_s]
  [VVMC_RRWhlSpdSlideRate_pct] -> VVMC_RRWhlSpdSlideRate_pct/1
  VINP_BrkPedalPos_pct/1 -> [VINP_BrkPedalPos_pct]
  [VVMC_LFWhlSpdSlideRate_pct] -> VVMC_LFWhlSpdSlideRate_pct/1
  VTQD_EquivAccPedalSWSta_flg/1 -> [VTQD_EquivAccPedalSWSta_flg]
  [VVMC_ActRRSlideRate_pct] -> VVMC_ActRRSlideRate_pct/1
  [VVMC_RF4WhlSpdSlideRate_pct] -> VVMC_RF4WhlSpdSlideRate_pct/1
  VTQD_AfterAvailableTqDemFr_Nm/1 -> [VTQD_AfterAvailableTqDemFr_Nm]
  VINP_BrkSwSta_flg/1 -> [VINP_BrkSwSta_flg]

== system vmc/VMC/VMC/SpeedArbitration ==
  VVMC_VMCCCCtrlAvail_flg : Inport
  VVMC_VMCMSACtrlAvail_flg : Inport  Port=2
  VVMC_VMCACCCtrlAvail_flg : Inport  Port=3
  VVMC_VMCAEBCtrlAvail_flg : Inport  Port=4
  VINP_ADASAEBReq_enum : Inport  Port=5
  VINP_ADASAEBSta_enum : Inport  Port=6
  VDSC_DISCSta_enum : Inport  Port=7
  VINP_ADASACCSta_enum : Inport  Port=8
  VVMC_CCCtrlSta_enum : Inport  Port=9
  VVMC_MSACtrlSta_enum : Inport  Port=10
  VDSC_DISCTargetSpd_kph : Inport  Port=11
  VVMC_FeatSetSpdForCalcu_kph : Inport  Port=12
  VDSC_DISCTurn_flg : Inport  Port=13
  VVMC_MeterIndSpeedForCalcu_kph : Inport  Port=14
  VVMC_VehicleSpeed_kph : Inport  Port=15
  VDSC_AccDecResp_flg : Inport  Port=16
  VDSC_AutoTurnMode_flg : Inport  Port=17
  VVMC_AntiSpdLimSpdEn_flg : Inport  Port=18
  VVMC_AntiLimitSpd_kph : Inport  Port=19
  VDSC_PreACC_flg : Inport  Port=20
  AND : Logic  AllPortsSameDT=off  OutDataTypeStr=boolean
  AND1 : Logic  AllPortsSameDT=off  OutDataTypeStr=boolean
  Cast To Single : DataTypeConversion  OutDataTypeStr=uint8
  Cast To Single1 : DataTypeConversion  OutDataTypeStr=uint8
  Cast To Single2 : DataTypeConversion  OutDataTypeStr=single
  Cast To Single3 : DataTypeConversion  OutDataTypeStr=single
  Cast To Single4 : DataTypeConversion  OutDataTypeStr=single
  Constant : Constant  Value=KVMC_ExternalCtrlSW_flg
  Constant1 : Constant  Value=KVMC_ExternalCtrlSW_flg
  Constant11 : Constant  Value=KVMC_DISCDecCtrlTest_flg
  Constant12 : Constant  Value=ENUM_DISCSTA_ACTIVE
  Constant13 : Constant  Value=HUNDRED
  Constant14 : Constant  Value=KVMC_DISCDecCtrlTest_flg
  Constant15 : Constant  Value=ENUM_DISCSTA_ACTIVE
  Constant16 : Constant  Value=HUNDRED
  Constant2 : Constant  Value=KVMC_ExternalCtrlSW_flg
  Constant3 : Constant  Value=KVMC_ExternalCtrlSta_enum
  Constant4 : Constant  Value=KVMC_ExternalSpeedTarget_kph
  Constant5 : Constant  Value=KVMC_ExternalCtrlAGSV_flg
  Constant6 : Constant  Value=KVMC_AutoTurnJerkHiGain_pct
  Constant7 : Constant  Value=KVMC_AutoTurnLimitHiGain_pct
  Constant8 : Constant  Value=ENUM_FEATSTACFM_MSA
  Constant9 : Constant  Value=ENUM_FEATSTACFM_MSA
  Divide : Product  Inputs=**
  Divide1 : Product  Inputs=**
  Feature Arbitration : Subsystem
  Feature Status Confirm : Subsystem
  OR : Logic  Operator=OR  Inputs=3  AllPortsSameDT=off  OutDataTypeStr=boolean
  OR1 : Logic  Operator=OR  Inputs=3  AllPortsSameDT=off  OutDataTypeStr=boolean
  Relational Operator : RelationalOperator  Operator===  OutDataTypeStr=boolean  RndMeth=Simplest
  Relational Operator1 : RelationalOperator  Operator===  OutDataTypeStr=boolean  RndMeth=Simplest
  Response Gain : Subsystem
  Round : Rounding  Operator=round
  Switch{,1..9} (10 alike) : Switch  Criteria=u2 > Threshold
  VVMC_FeatArbitrSta_enum : Outport
  VVMC_FeatReqSpd_kph : Outport  Port=2
  VVMC_JerkPCT_pct : Outport  Port=3
  VVMC_LimitPCT_pct : Outport  Port=4
  wires:
  [VDSC_PreACC_flg] -> Feature Arbitration/4(VDSC_PreACC_flg)
  [VDSC_PreACC_flg] -> Feature Status Confirm/11(VDSC_PreACC_flg)
  Switch8/1 -> [VVMC_JerkPCT_pct]  "VVMC_JerkPCT_pct"
  AND/1 -> Switch8/2
  OR/1 -> AND/1
  [VDSC_AutoTurnMode_flg] -> OR/3
  Constant11/1 -> AND/2
  Constant12/1 -> Relational Operator/2
  [VDSC_PreACC_flg] -> OR/1
  Constant13/1 -> Switch8/1
  Relational Operator/1 -> OR/2
  [VDSC_DISCSta_enum] -> Relational Operator/1
  Switch9/1 -> [VVMC_LimitPCT_pct]  "VVMC_LimitPCT_pct"
  Constant14/1 -> AND1/2
  Constant16/1 -> Switch9/1
  [VDSC_AutoTurnMode_flg] -> OR1/3
  [VDSC_DISCSta_enum] -> Relational Operator1/1
  Constant15/1 -> Relational Operator1/2
  OR1/1 -> AND1/1
  [VDSC_PreACC_flg] -> OR1/1
  Relational Operator1/1 -> OR1/2
  AND1/1 -> Switch9/2
  VDSC_PreACC_flg/1 -> [VDSC_PreACC_flg]
  VVMC_AntiLimitSpd_kph/1 -> [VVMC_AntiLimitSpd_kph]
  [VDSC_DISCTargetSpd_kph] -> Response Gain/7(VDSC_DISCTargetSpd_kph)
  [VVMC_AntiLimitSpd_kph] -> Switch7/1
  Cast To Single2/1 -> Switch7/3
  [VVMC_AntiSpdLimSpdEn_flg] -> Switch7/2
  Cast To Single1/1 -> Switch6/3
  [VVMC_AntiSpdLimSpdEn_flg] -> Switch6/2
  Constant9/1 -> Switch6/1
  Constant8/1 -> Switch5/1
  Cast To Single/1 -> Switch5/3
  [VVMC_AntiSpdLimSpdEn_flg] -> Switch5/2
  VVMC_AntiSpdLimSpdEn_flg/1 -> [VVMC_AntiSpdLimSpdEn_flg]
  [VDSC_AutoTurnMode_flg] -> Response Gain/6(VDSC_AutoTurnMode_flg)
  VDSC_AutoTurnMode_flg/1 -> [VDSC_AutoTurnMode_flg]
  [VDSC_AccDecResp_flg] -> Switch4/2
  Cast To Single4/1 -> Switch4/3, Divide1/2
  Constant7/1 -> Divide1/1
  Divide1/1 -> Switch4/1
  Divide/1 -> Switch3/1
  Constant6/1 -> Divide/1
  Cast To Single3/1 -> Divide/2, Switch3/3
  [VDSC_AccDecResp_flg] -> Switch3/2
  VDSC_AccDecResp_flg/1 -> [VDSC_AccDecResp_flg]
  [VDSC_DISCTurn_flg] -> Switch2/3
  Constant/1 -> Switch/2
  Constant4/1 -> Switch1/1
  Constant2/1 -> Switch2/2
  Constant3/1 -> Switch/1
  [VDSC_DISCTargetSpd_kph] -> Switch1/3
  Constant5/1 -> Switch2/1
  Constant1/1 -> Switch1/2
  [VDSC_DISCSta_enum] -> Switch/3
  Switch1/1 -> Feature Arbitration/2(VDSC_DISCTargetSpd_kph)
  VINP_ADASAEBSta_enum/1 -> [VINP_ADASAEBSta_enum]
  VDSC_DISCSta_enum/1 -> [VDSC_DISCSta_enum]
  VINP_ADASACCSta_enum/1 -> [VINP_ADASACCSta_enum]
  VVMC_CCCtrlSta_enum/1 -> [VVMC_CCCtrlSta_enum]
  VVMC_MSACtrlSta_enum/1 -> [VVMC_MSACtrlSta_enum]
  VDSC_DISCTargetSpd_kph/1 -> [VDSC_DISCTargetSpd_kph]
  VVMC_FeatSetSpdForCalcu_kph/1 -> [VVMC_FeatSetSpdForCalcu_kph]
  VDSC_DISCTurn_flg/1 -> [VDSC_DISCTurn_flg]
  [VINP_ADASAEBSta_enum] -> Feature Status Confirm/5(VINP_ADASAEBSta_enum)
  Switch/1 -> Feature Status Confirm/6(VDSC_DISCSta_enum)
  [VINP_ADASACCSta_enum] -> Feature Status Confirm/7(VINP_ADASACCSta_enum)
  [VVMC_CCCtrlSta_enum] -> Feature Status Confirm/8(VVMC_CCCtrlSta_enum)
  [VVMC_MSACtrlSta_enum] -> Feature Status Confirm/9(VVMC_MSACtrlSta_enum)
  Feature Status Confirm/1(VVMC_FeatStaConfirm_enum) -> Cast To Single/1
  [VVMC_FeatStaConfirm_enum] -> Feature Arbitration/1(VVMC_FeatStaConfirm_enum)
  [VVMC_FeatSetSpdForCalcu_kph] -> Feature Arbitration/3(VVMC_FeatSetSpdForCalcu_kph)
  Feature Arbitration/1(VVMC_FeatArbitrSta_enum) -> Cast To Single1/1
  Feature Arbitration/2(VVMC_FeatReqSpd_kph) -> Round/1
  [VVMC_FeatArbitrSta_enum] -> VVMC_FeatArbitrSta_enum/1
  [VVMC_FeatReqSpd_kph] -> VVMC_FeatReqSpd_kph/1
  Switch2/1 -> Response Gain/1(VDSC_DISCTurn_flg)
  [VVMC_FeatArbitrSta_enum] -> Response Gain/2(VVMC_FeatArbitrSta_enum)
  Response Gain/2(VVMC_LimitPCT_pct) -> Cast To Single4/1
  Response Gain/1(VVMC_JerkPCT_pct) -> Cast To Single3/1
  [VVMC_LimitPCT_pct] -> VVMC_LimitPCT_pct/1
  [VVMC_JerkPCT_pct] -> VVMC_JerkPCT_pct/1
  Switch5/1 -> [VVMC_FeatStaConfirm_enum]  "VVMC_FeatStaConfirm_enum"
  Switch6/1 -> [VVMC_FeatArbitrSta_enum]  "VVMC_FeatArbitrSta_enum"
  Switch7/1 -> [VVMC_FeatReqSpd_kph]  "VVMC_FeatReqSpd_kph"
  Switch3/1 -> Switch8/3
  Switch4/1 -> Switch9/3
  VVMC_VMCACCCtrlAvail_flg/1 -> [VVMC_VMCACCCtrlAvail_flg]
  VVMC_VMCAEBCtrlAvail_flg/1 -> [VVMC_VMCAEBCtrlAvail_flg]
  [VVMC_VMCACCCtrlAvail_flg] -> Feature Status Confirm/4(VVMC_VMCACCCtrlAvail_flg)
  [VVMC_VMCAEBCtrlAvail_flg] -> Feature Status Confirm/3(VVMC_VMCAEBCtrlAvail_flg)
  VVMC_VMCMSACtrlAvail_flg/1 -> [VVMC_VMCMSACtrlAvail_flg]
  VVMC_VMCCCCtrlAvail_flg/1 -> [VVMC_VMCCCCtrlAvail_flg]
  [VVMC_VMCMSACtrlAvail_flg] -> Feature Status Confirm/2(VVMC_VMCMSACtrlAvail_flg)
  [VVMC_VMCCCCtrlAvail_flg] -> Feature Status Confirm/1(VVMC_VMCCCCtrlAvail_flg)
  VINP_ADASAEBReq_enum/1 -> [VINP_ADASAEBReq_enum]
  [VINP_ADASAEBReq_enum] -> Feature Status Confirm/10(VINP_ADASAEBReq_enum)
  Round/1 -> Cast To Single2/1
  VVMC_MeterIndSpeedForCalcu_kph/1 -> [VVMC_MeterIndSpeedForCalcu_kph]
  [VVMC_MeterIndSpeedForCalcu_kph] -> Response Gain/4(VVMC_MeterIndSpeedForCalcu_kph)
  [VVMC_FeatReqSpd_kph] -> Response Gain/3(VVMC_FeatReqSpd_kph)
  VVMC_VehicleSpeed_kph/1 -> [VVMC_VehicleSpeed_kph]
  [VVMC_VehicleSpeed_kph] -> Response Gain/5(VVMC_VehicleSpeed_kph)

== system vmc/VMC/VMC/SpeedCalculation ==
  VINP_MeterIndVehSpeed_kph : Inport
  VINP_Distanceunit_flg : Inport  Port=2
  VINP_VehSpeed_kph : Inport  Port=3
  VTQD_VehActSpd_kph : Inport  Port=4
  VDDM_ESC1Err_flg : Inport  Port=5
  VDDM_ESC5Err_flg : Inport  Port=6
  task_time_s : Inport  Port=7
  function : TriggerPort  TriggerType=function-call  VariantControl=(inherit)
  Add4 : Sum
  Add8 : Sum
  Cast To Single1 : DataTypeConversion  OutDataTypeStr=uint8
  Cast To Single{2..3,6..7,10..12} (7 alike) : DataTypeConversion  OutDataTypeStr=single
  Cast To Single13 : DataTypeConversion  OutDataTypeStr=uint8
  Constant1 : Constant  Value=KVMC_MeterSpdRoundSW_flg
  Constant10 : Constant  Value=KVMC_MeterSpdSourceSW_flg
  Constant11 : Constant  Value=KPH2MPH
  Constant16 : Constant  Value=KVMC_Veh2MeterSpdFactor_enum
  Constant19 : Constant  Value=KPH2MPH
  Constant2 : Constant  Value=KVMC_MeterSpdRoundSW_flg
  Constant23 : Constant  Value=KVMC_MeterSpdBWFilter_raw32
  Constant28 : Constant  Value=KVMC_Veh2MeterSpdLoFactor_enum
  Constant3 : Constant  Value=ONE_INT
  Constant4 : Constant  Value=ONE_INT
  Constant5 : Constant  Value=KVMC_MeterSpdRollAveLevel_enum
  Constant6 : Constant  Value=256
  Constant7 : Constant  Value=ZERO_FLOAT
  Constant8 : Constant  Value=KVMC_Veh2MeterSpdOffset_enum
  Constant9 : Constant  Value=256
  Divide{,2,5,8} (4 alike) : Product  Inputs=**
  FirstOrderFilter6 : hcu_lib/Basic_Blocks/FirstOrderFilter
  Min : MinMax  Function=max  Inputs=2
  OR : Logic  Operator=OR  AllPortsSameDT=off  OutDataTypeStr=boolean
  OR1 : Logic  Operator=OR  AllPortsSameDT=off  OutDataTypeStr=boolean
  Relational Operator : RelationalOperator  Operator=>  OutDataTypeStr=boolean  RndMeth=Simplest
  Relational Operator1 : RelationalOperator  Operator=>  OutDataTypeStr=boolean  RndMeth=Simplest
  RollingAverage : Stateflow chart  TreatAsAtomicUnit=on
  Round : Rounding
  Round1 : Rounding  Operator=round
  Round2 : Rounding
  Round3 : Rounding  Operator=round
  Switch : Switch  Criteria=u2 > Threshold
  Switch1 : Switch  Criteria=u2 > Threshold  Threshold=KVMC_Veh2MeterSpdLoBdy_kph
  Switch2 : Switch  Criteria=u2 > Threshold
  Switch3 : Switch  Criteria=u2 > Threshold
  u2 > 0 (1) : Switch  Criteria=u2 > Threshold
  u2 > 0 (1)1 : Switch  Criteria=u2 > Threshold
  u2 > 0 (1)2 : Switch  Criteria=u2 > Threshold
  VVMC_MeterIndSpeed_raw32 : Outport
  VVMC_VehicleSpeed_mph : Outport  Port=2
  VVMC_VehicleSpeed_kph : Outport  Port=3
  VVMC_MeterIndSpeedForCalcu_kph : Outport  Port=4
  wires:
  Constant10/1 -> Switch3/2
  Switch3/1 -> Switch/3
  [VTQD_VehActSpd_kph] -> Switch2/1
  [VINP_VehSpeed_kph] -> Switch2/3
  [VINP_VehSpeed_kph] -> Relational Operator1/1
  Relational Operator1/1 -> OR1/1
  Constant9/1 -> Relational Operator1/2
  [VDDM_ESC1Err_flg] -> OR1/2
  OR1/1 -> Switch2/2
  [VINP_MeterIndVehSpeed_kph] -> Switch3/3
  OR/1 -> Switch/2
  [VVMC_VehicleSpeed_kph] -> Divide5/2, Divide8/1, Switch1/2
  Divide5/1 -> Add4/2
  Constant16/1 -> Divide5/1
  Divide8/1 -> Switch1/3
  Add4/1 -> Switch1/1
  Constant8/1 -> Add4/1
  Switch1/1 -> Switch/1, Switch3/1
  Constant28/1 -> Divide8/2
  [VDDM_ESC5Err_flg] -> OR/2
  Relational Operator/1 -> OR/1
  Constant6/1 -> Relational Operator/2
  [VINP_MeterIndVehSpeed_kph] -> Relational Operator/1
  VDDM_ESC5Err_flg/1 -> [VDDM_ESC5Err_flg]
  VDDM_ESC1Err_flg/1 -> [VDDM_ESC1Err_flg]
  VTQD_VehActSpd_kph/1 -> [VTQD_VehActSpd_kph]
  Constant3/1 -> Min/2
  Min/1 -> RollingAverage/1(KVMC_RollAveLevel_enum)
  Cast To Single1/1 -> Min/1
  Cast To Single11/1 -> RollingAverage/2(ZERO_FLOAT)
  Cast To Single13/1 -> RollingAverage/3(ONE_INT)
  Cast To Single12/1 -> RollingAverage/4(VINP_RawData_kph)
  Constant7/1 -> Cast To Single11/1
  Constant4/1 -> Cast To Single13/1
  Switch/1 -> Cast To Single12/1
  Constant5/1 -> Cast To Single1/1
  RollingAverage/1(VVMC_RollAve_kph) -> Cast To Single3/1
  Round3/1 -> u2 > 0 (1)2/1
  Constant2/1 -> u2 > 0 (1)2/2
  Round2/1 -> u2 > 0 (1)2/3
  Round1/1 -> u2 > 0 (1)1/1
  Round/1 -> u2 > 0 (1)1/3
  Constant1/1 -> u2 > 0 (1)1/2
  Cast To Single3/1 -> FirstOrderFilter6/1
  Constant23/1 -> Add8/2
  Add8/1 -> FirstOrderFilter6/3
  [task_time_s] -> FirstOrderFilter6/2, Add8/1
  [VVMC_VehicleSpeed_mph] -> VVMC_VehicleSpeed_mph/1
  Cast To Single10/1 -> [VVMC_VehicleSpeed_kph]  "VVMC_VehicleSpeed_kph"
  Divide2/1 -> [VVMC_VehicleSpeed_mph]  "VVMC_VehicleSpeed_mph"
  VINP_MeterIndVehSpeed_kph/1 -> [VINP_MeterIndVehSpeed_kph]
  Cast To Single7/1 -> Divide/1
  Switch2/1 -> Cast To Single2/1, Cast To Single10/1
  [VVMC_MeterSpdRollAve_kph] -> Round3/1, Round2/1, u2 > 0 (1)/3, Cast To Single7/1  "VVMC_MeterSpdRollAve_kph"
  Divide/1 -> u2 > 0 (1)/1
  VINP_VehSpeed_kph/1 -> [VINP_VehSpeed_kph]
  u2 > 0 (1)1/1 -> [VVMC_MeterIndSpeed_raw32]  "VVMC_MeterIndSpeed_raw32"
  [VVMC_MeterIndSpeedForCalcu_kph] -> VVMC_MeterIndSpeedForCalcu_kph/1
  Cast To Single2/1 -> Divide2/1
  Constant11/1 -> Divide2/2
  Cast To Single6/1 -> Round/1, Round1/1
  [VVMC_VehicleSpeed_kph] -> VVMC_VehicleSpeed_kph/1
  u2 > 0 (1)2/1 -> [VVMC_MeterIndSpeedForCalcu_kph]  "VVMC_MeterIndSpeedForCalcu_kph"
  Constant19/1 -> Divide/2
  [VVMC_MeterIndSpeed_raw32] -> VVMC_MeterIndSpeed_raw32/1
  FirstOrderFilter6/1 -> [VVMC_MeterSpdRollAve_kph]  "VVMC_MeterSpdRollAve_kph"
  [VINP_Distanceunit_flg] -> u2 > 0 (1)/2
  VINP_Distanceunit_flg/1 -> [VINP_Distanceunit_flg]
  u2 > 0 (1)/1 -> Cast To Single6/1
  task_time_s/1 -> [task_time_s]
